simulink model "Robust_Control"  (R2023b)
settings: Solver=ode1  StartTime=0.0  StopTime=50  FixedStep=Tc  RelTol=1e-3
values from neighbouring files (symbols this model uses):
  Tc = 0.001    [scara_parameters.m]
undefined symbols (not defined in the file or in its folder): D, K_D_Rob, K_P_Rob, mload, Q, q0, rhovers
settings Model: Creator=emman  LastModifiedBy=emman

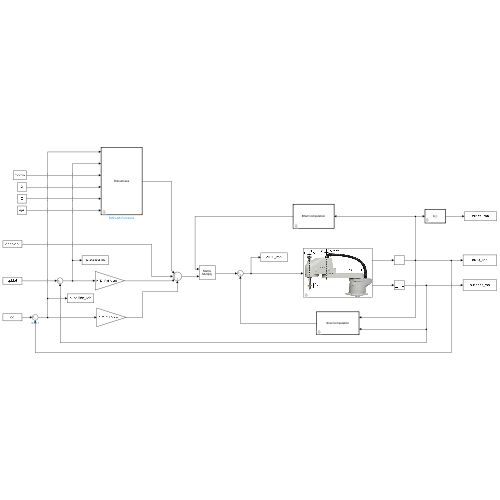
[thumbnail: Simulink's stored preview of the top-level diagram]
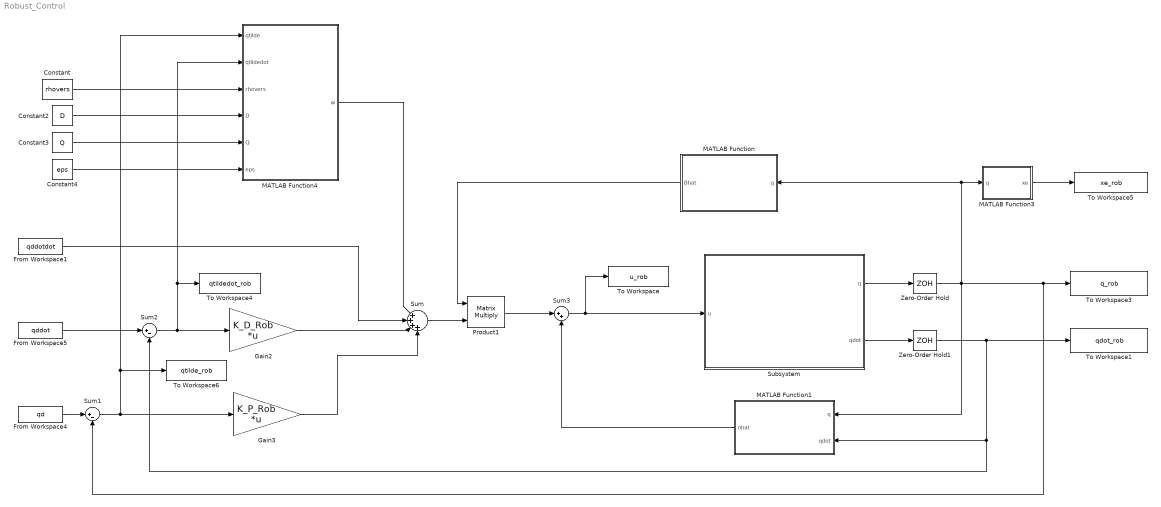
== system Robust_Control ==
  Constant : Constant  Value=rhovers
  Constant2 : Constant  Value=D
  Constant3 : Constant  Value=Q
  Constant4 : Constant  Value=eps
  From Workspace1 : FromWorkspace  VariableName=qddotdot  SampleTime=Tc
  From Workspace4 : FromWorkspace  VariableName=qd  SampleTime=Tc
  From Workspace5 : FromWorkspace  VariableName=qddot  SampleTime=Tc
  Gain2 : Gain  Gain=K_D_Rob  Multiplication=Matrix(K*u) (u vector)
  Gain3 : Gain  Gain=K_P_Rob  Multiplication=Matrix(K*u) (u vector)
  MATLAB Function : MATLAB Function  TreatAsAtomicUnit=on
  MATLAB Function1 : MATLAB Function  TreatAsAtomicUnit=on
  MATLAB Function3 : MATLAB Function  TreatAsAtomicUnit=on
  MATLAB Function4 : MATLAB Function  TreatAsAtomicUnit=on
  Product1 : Product  Multiplication=Matrix(*)
  Subsystem : Subsystem
      mask Display: image('SCARA.png');
  Sum : Sum  Inputs=|++++
  Sum1 : Sum  Inputs=|+-
  Sum2 : Sum  Inputs=|+-
  Sum3 : Sum  Inputs=|++
  To Workspace : ToWorkspace  VariableName=u_rob  SaveFormat=Structure With Time  SampleTime=-1
  To Workspace1 : ToWorkspace  VariableName=qdot_rob  SaveFormat=Structure With Time  SampleTime=-1
  To Workspace3 : ToWorkspace  VariableName=q_rob  SaveFormat=Structure With Time  SampleTime=-1
  To Workspace4 : ToWorkspace  VariableName=qtildedot_rob  SaveFormat=Structure With Time  SampleTime=-1
  To Workspace5 : ToWorkspace  VariableName=xe_rob  SaveFormat=Structure With Time  SampleTime=-1
  To Workspace6 : ToWorkspace  VariableName=qtilde_rob  SaveFormat=Structure With Time  SampleTime=-1
  Zero-Order Hold : ZeroOrderHold  SampleTime=Tc
  Zero-Order Hold1 : ZeroOrderHold  SampleTime=Tc
  wires:
  From Workspace4/1 -> Sum1/1
  Sum1/1 -> Gain3/1, MATLAB Function4/1(qtilde), To Workspace6/1
  Sum/1 -> Product1/2
  From Workspace5/1 -> Sum2/1
  Sum2/1 -> MATLAB Function4/2(qtildedot), To Workspace4/1, Gain2/1
  Gain3/1 -> Sum/4
  Gain2/1 -> Sum/3
  From Workspace1/1 -> Sum/2
  Constant4/1 -> MATLAB Function4/6(eps)
  Constant3/1 -> MATLAB Function4/5(Q)
  Constant2/1 -> MATLAB Function4/4(D)
  Constant/1 -> MATLAB Function4/3(rhovers)
  MATLAB Function4/1(w) -> Sum/1
  MATLAB Function/1(Bhat) -> Product1/1
  Product1/1 -> Sum3/1
  MATLAB Function1/1(nhat) -> Sum3/2
  Zero-Order Hold/1 -> Sum1/2, To Workspace3/1, MATLAB Function1/1(q), MATLAB Function3/1(q), MATLAB Function/1(q)
  Subsystem/1(q) -> Zero-Order Hold/1
  Subsystem/2(qdot) -> Zero-Order Hold1/1
  Sum3/1 -> Subsystem/1(u), To Workspace/1
  Zero-Order Hold1/1 -> To Workspace1/1, MATLAB Function1/2(qdot), Sum2/2
  MATLAB Function3/1(xe) -> To Workspace5/1

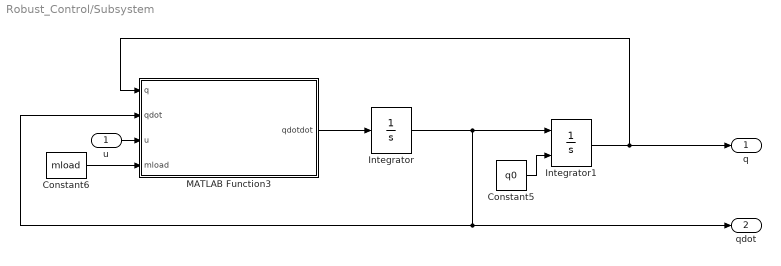
== system Robust_Control/Subsystem ==
  u : Inport
  Constant5 : Constant  Value=q0
  Constant6 : Constant  Value=mload
  Integrator : Integrator  InitialCondition=[0 0 0 0]'
  Integrator1 : Integrator  InitialConditionSource=external
  MATLAB Function3 : MATLAB Function  TreatAsAtomicUnit=on
  q : Outport
  qdot : Outport  Port=2
  wires:
  Constant6/1 -> MATLAB Function3/4(mload)
  Integrator/1 -> Integrator1/1, qdot/1, MATLAB Function3/2(qdot)
  u/1 -> MATLAB Function3/3(u)
  Integrator1/1 -> q/1, MATLAB Function3/1(q)
  MATLAB Function3/1(qdotdot) -> Integrator/1
  Constant5/1 -> Integrator1/2

== matlab function Robust_Control/MATLAB Function1 ==
  data: q input; nhat output; qdot input
function nhat = nhatComputation(q,qdot)
    
    %m
    a1 = 0.5;
    a2 = 0.5;
    
    %m
    l1 = 0.25;
    l2 = 0.25;
    
    %kg
    ml1 = 20;
    ml2 = 20;
    ml3 = 10;
    
    %rad/m
    kr1 = 1;
    kr2 = 1;
    kr3 = 50;
    kr4 = 20;
    
    
    %N*m*s/rad
    Fm1 = 0.00005;
    Fm2 = 0.00005;
    Fm3 = 0.01;
    Fm4 = 0.005;
    
    %NON-Linear Terms

    %Christoffel Symbols
    c = zeros(4,4,4);
    
    %c_ijk = 1/2*(db_ij/dq_k + db_ik/dq_j - db_jk/dq_i)
    %For Example: c_112 = 1/2*(db_11/dq_2 + db_12/dq_1 - db_12/dq_1) =
    % = 1/2 * db_11/dq_2
    %Christoffel Symbols Properties:
    %c_iii = 0 since db_ii/dq_i = 0 for all i
    %c_ijk = c_ikj
    %Additionally b_ji = b_ij

    %Using the file InertiaMatrix.m in this folder it is possible to
    %visualize the matrix B(4x4) and the various b_11, b_12, b_21 and b_22
    %with the command (B(1,1), B(1,2), B(2,1) and B(2,2))

    c(1,1,2) = 1/2*(-2*a1*a2*ml3*sin(q(2))-2*a1*l2*ml2*sin(q(2)) + 0 ); 
    c(1,2,1) = c(1,1,2);
    
    %c_211 = 1/2*(db_21/dq_1 + db_21/dq_1 - db_11/dq_2) = -1/2 * db_11/dq_2
    %So c_211 = -c_112
    c(2,1,1) = -c(1,1,2);

    %c_122 = 1/2*(db_12/dq_2 + db_12/dq_2 - b_22/dq_1) = db_12/dq_2
    c(1,2,2) = -a1*a2*ml3*sin(q(2)) - a1*l2*ml2*sin(q(2));
    %It is possible to note that also c(1,2,2) = c(1,1,2)

    %c_212 = c_221 = 1/2*(db_21/dq_2 + db_22/dq_1 - db_12/dq_2) = 0
    %The other Christoffel Symbols are all nulls because B does not depend
    %on q(3) and q(4)
    C=zeros(4,4);

    %c(q,qdot)=C(q,qdot)*qdot
    %c_ik = c_ijk(q)qdot_j
    %c_ik is the ik element of the matrix C

    for i=1:4
        for j=1:4
            for k=1:4
                C(i,k)= C(i,k)+c(i,j,k)*qdot(j);    %C(i,k) in the second term is superfluous
            end
        end
    end

    %Gravitational Term
    g = [0 0 ml3*9.81 0]';

    %Vicous Friction Term
    %To convert from the motor side to the joint side,
    % it is necessary to multiply by the transmission ratio.
    Fv = diag([kr1^2*Fm1 kr2^2*Fm2 kr3^2*Fm3 kr4^2*Fm4]);
    
    %It is applied an intentional neglection of the C*qdot term
    %nhat = C*qdot + Fv*qdot + g;
    nhat = Fv*qdot + g;
end

== matlab function Robust_Control/MATLAB Function ==
  data: q input; Bhat output
function Bhat = BhatComputation(q)
      
    B = BComputation(q);
    
    Bhat = diag([B(1,1) B(2,2) B(3,3) B(4,4)]);
    
end

== matlab function Robust_Control/MATLAB Function3 ==
  data: q input; xe output
function xe = DirKin(q)

    xe = k(q);

end

== matlab function Robust_Control/Subsystem/MATLAB Function3 ==
  data: q input; qdotdot output; qdot input; u input; mload input
function qdotdot = DirectDynamic(q,qdot,u,mload)
    
    %m
    a1 = 0.5;
    a2 = 0.5;
    l1 = 0.25;
    l2 = 0.25;
    
    %kg
    ml1 = 20;
    ml2 = 20;
    ml3 = 10;
    
    %rad/m
    kr1 = 1;
    kr2 = 1;
    kr3 = 50;
    kr4 = 20;
        
    %N*m*s/rad
    Fm1 = 0.00005;
    Fm2 = 0.00005;
    Fm3 = 0.01;
    Fm4 = 0.005;
    
    B = BComputation(q);

    %Christoffel Symbols
    c = zeros(4,4,4);
    
    %c_ijk = 1/2*(db_ij/dq_k + db_ik/dq_j - db_jk/dq_i)
    %For Example: c_112 = 1/2*(db_11/dq_2 + db_12/dq_1 - db_12/dq_1) =
    % = 1/2 * db_11/dq_2
    %Christoffel Symbols Properties:
    %c_iii = 0 since db_ii/dq_i = 0 for all i
    %c_ijk = c_ikj
    %Additionally b_ji = b_ij

    %Using the file InertiaMatrix.m in this folder it is possible to
    %visualize the matrix B(4x4) and the various b_11, b_12, b_21 and b_22
    %with the command (B(1,1), B(1,2), B(2,1) and B(2,2))

    c(1,1,2) = 1/2*(-2*a1*a2*ml3*sin(q(2))-2*a1*l2*ml2*sin(q(2)) + 0 ); 
    c(1,2,1) = c(1,1,2);
    
    %c_211 = 1/2*(db_21/dq_1 + db_21/dq_1 - db_11/dq_2) = -1/2 * db_11/dq_2
    %So c_211 = -c_112
    c(2,1,1) = -c(1,1,2);

    %c_122 = 1/2*(db_12/dq_2 + db_12/dq_2 - b_22/dq_1) = db_12/dq_2
    c(1,2,2) = -a1*a2*ml3*sin(q(2)) - a1*l2*ml2*sin(q(2));
    %It is possible to note that also c(1,2,2) = c(1,1,2)

    %c_212 = c_221 = 1/2*(db_21/dq_2 + db_22/dq_1 - db_12/dq_2) = 0
    %The other Christoffel Symbols are all nulls because B does not depend
    %on q(3) and q(4)
    C=zeros(4,4);

    %c(q,qdot)=C(q,qdot)*qdot
    %c_ik = c_ijk(q)qdot_j
    %c_ik is the ik element of the matrix C

    for i=1:4
        for j=1:4
            for k=1:4
                C(i,k)= C(i,k)+c(i,j,k)*qdot(j);    %C(i,k) in the second term is superfluous
            end
        end
    end
    
    %Gravity of link 3 (ml3) and load (mload)
    g = [0 0 9.81*(ml3+mload) 0]';

    %Viscous Friction
    Fv=diag([kr1^2*Fm1 kr2^2*Fm2 kr3^2*Fm3 kr4^2*Fm4]);

    %Acceleration
    qdotdot = inv(B)*(u-C*qdot-Fv*qdot-g);

end

== matlab function Robust_Control/MATLAB Function4 ==
  data: qtilde input; w output; qtildedot input; rhovers input; D input; Q input; eps input
function w = Robustness(qtilde,qtildedot,rhovers,D,Q,eps)

    % w = rho/||z|| * z if ||z||>=eps
    % w = rho/eps * z if ||z||<eps
    zita = [qtilde;qtildedot];
    z = D'*Q*zita;

    if norm(z) >= eps
        w = rhovers*(z/norm(z));
    else
        w = rhovers*(z/eps);
    end

end
